simulink model "sedemo_async_clocks"  (Simulink 7.5)
settings: Solver=VariableStepDiscrete  StartTime=0.0  StopTime=10.0  MaxStep=inf  RelTol=1e-3
libraries: simulink x4, simeventstranslate1 x2, simeventsinfo x1, simeventssink1 x1
settings Model: Creator=The MathWorks Inc.  ExtModeAutoUpdateStatusClock=off
settings DataIOCC: SaveOutput=off  SaveTime=off
settings OptimizationCC: InitFltsAndDblsToZero=on
settings DebuggingCC: ReadBeforeWriteMsg=DisableAll  WriteAfterWriteMsg=DisableAll  WriteAfterReadMsg=DisableAll  AlgebraicLoopMsg=error  SolverPrmCheckMsg=none  StrictBusMsg=Warning
settings SimEventsCC: propDiagAttribOutput=1  propDiagFcnCallOutput=1  propDiagStatOutput=0

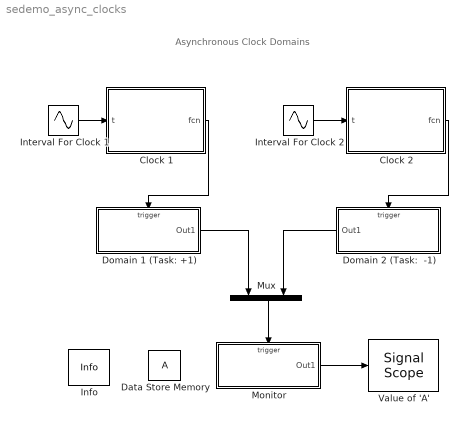
== system sedemo_async_clocks ==
  note: Asynchronous Clock Domains
  Clock 1 : Subsystem
  Clock 2 : Subsystem
  Data Store Memory : DataStoreMemory  DataStoreName=A  ReadBeforeWriteMsg=warning  WriteAfterWriteMsg=warning  WriteAfterReadMsg=warning  OutDataType=sfix(16)  OutScaling=2^0
  Domain 1 (Task: +1) : Subsystem  TreatAsAtomicUnit=on
  Domain 2 (Task:  -1) : Subsystem  TreatAsAtomicUnit=on
  Info : simeventsinfo/Info  SystemSampleTime=-1
  Interval For Clock 1 : Sin  Amplitude=-0.0001  Bias=.01  Frequency=1  Phase=pi/2  Samples=10  SampleTime=0  Offset=0
  Interval For Clock 2 : Sin  Amplitude=0.0001  Bias=.01  Frequency=1  Phase=pi/2  Samples=10  SampleTime=0  Offset=0
  Monitor : Subsystem  TreatAsAtomicUnit=on
      settings: PropExecContextOutsideSubsystem=on
  Mux : Mux  Inputs=2
  Value of 'A' : simeventssink1/Signal Scope  Priority=1  SystemSampleTime=-1  PlotType=Stair  InputType=Signal  NumInputs=1  AttributeNameY=Count  XInputOptionSignal=Event time  XInputOptionEntity=Event time  AttributeNameX=Count  EnableEntityOutport=on  XMin=-0.0999478213651573  XMax=10.0947299578809  XLimitExceededOption=Stretch axis limits  YLimitExceededOption=Stretch axis limits  AxisGrid=on  AxisLegend=off  LineDisables=""  LineColors=b  LineStyles=-  LineMarkers=.  OpenScopeAtSimStart=on  Title=Value of 'A': Clocks with Independent Drift  YLabel='A'  XLabel=Time  FigurePosition=[425 745 445 220]  AxisZoom=off  DataStoreOption=Limited  DataPointsLimit=10000  StatNumberArrived=Off  ShowCountPlotted=off  ShowToolbar=on
      settings: YMin=-2.05  YMax=3.05
  wires:
  Interval For Clock 1/1 -> Clock 1/1(t)
  Clock 1/1(fcn) -> Domain 1 (Task: +1)/Trigger
  Interval For Clock 2/1 -> Clock 2/1(t)
  Clock 2/1(fcn) -> Domain 2 (Task:  -1)/Trigger
  Domain 1 (Task: +1)/1(Out1) -> Mux/1
  Domain 2 (Task:  -1)/1(Out1) -> Mux/2
  Mux/1 -> Monitor/Trigger
  Monitor/1(Out1) -> Value of 'A'/1

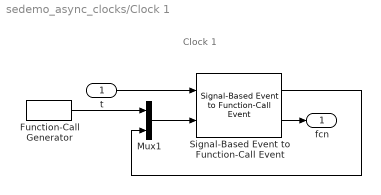
== system sedemo_async_clocks/Clock 1 ==
  note: Clock 1
  t : Inport
  Function-Call Generator : simulink/Ports & Subsystems/Function-Call Generator  sample_time=10000  numberOfIterations=1
  Mux1 : Mux  Inputs=2
  Signal-Based Event to Function-Call Event : simeventstranslate1/Signal-Based Event to Function-Call Event  Priority=1  SystemSampleTime=-1  GenerateFunctionCallUpon=Function call from port fcn  SignalEdgeOption=Rising  EnableE1Port=off  EnableF2Port=on  EnableE2Port=off  SpecifyEventPriority=on  PriorityFunctionCall=200  FunctionCallDelayFrom=Signal port t  DelayFunctionCall=0  StatNumberF1Calls=Off  StatNumberF2Calls=Off  MaskBlockType=none
  fcn : Outport
  wires:
  Mux1/1 -> Signal-Based Event to Function-Call Event/2
  Function-Call Generator/1 -> Mux1/1
  Signal-Based Event to Function-Call Event/1 -> Mux1/2
  t/1 -> Signal-Based Event to Function-Call Event/1
  Signal-Based Event to Function-Call Event/2 -> fcn/1

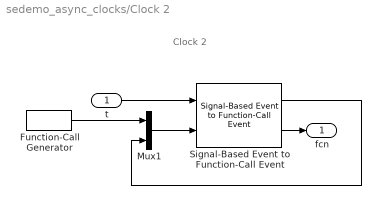
== system sedemo_async_clocks/Clock 2 ==
  note: Clock 2
  t : Inport
  Function-Call Generator : simulink/Ports & Subsystems/Function-Call Generator  sample_time=10000  numberOfIterations=1
  Mux1 : Mux  Inputs=2
  Signal-Based Event to Function-Call Event : simeventstranslate1/Signal-Based Event to Function-Call Event  Priority=1  SystemSampleTime=-1  GenerateFunctionCallUpon=Function call from port fcn  SignalEdgeOption=Rising  EnableE1Port=off  EnableF2Port=on  EnableE2Port=off  SpecifyEventPriority=on  PriorityFunctionCall=200  FunctionCallDelayFrom=Signal port t  DelayFunctionCall=0  StatNumberF1Calls=Off  StatNumberF2Calls=Off  MaskBlockType=none
  fcn : Outport
  wires:
  Mux1/1 -> Signal-Based Event to Function-Call Event/2
  Function-Call Generator/1 -> Mux1/1
  Signal-Based Event to Function-Call Event/1 -> Mux1/2
  t/1 -> Signal-Based Event to Function-Call Event/1
  Signal-Based Event to Function-Call Event/2 -> fcn/1

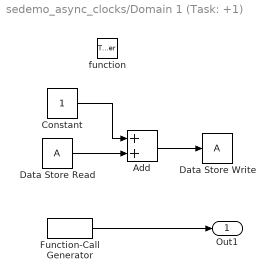
== system sedemo_async_clocks/Domain 1 (Task: +1) ==
  function : TriggerPort  TriggerType=function-call
  Add : Sum  OutDataType=sfix(16)  OutScaling=2^-10
  Constant : Constant  OutDataType=sfix(16)  OutScaling=2^0
  Data Store Read : DataStoreRead  DataStoreName=A  SampleTime=-1
  Data Store Write : DataStoreWrite  DataStoreName=A  SampleTime=-1
  Function-Call Generator : simulink/Ports & Subsystems/Function-Call Generator  sample_time=-1  numberOfIterations=1
  Out1 : Outport  OutDataType=sfix(16)  OutScaling=2^0
  wires:
  Add/1 -> Data Store Write/1
  Constant/1 -> Add/1
  Data Store Read/1 -> Add/2
  Function-Call Generator/1 -> Out1/1

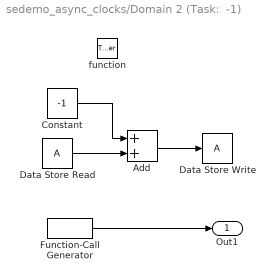
== system sedemo_async_clocks/Domain 2 (Task:  -1) ==
  function : TriggerPort  TriggerType=function-call
  Add : Sum  OutDataType=sfix(16)  OutScaling=2^-10
  Constant : Constant  Value=-1  OutDataType=sfix(16)  OutScaling=2^0
  Data Store Read : DataStoreRead  DataStoreName=A  SampleTime=-1
  Data Store Write : DataStoreWrite  DataStoreName=A  SampleTime=-1
  Function-Call Generator : simulink/Ports & Subsystems/Function-Call Generator  sample_time=-1  numberOfIterations=1
  Out1 : Outport  OutDataType=sfix(16)  OutScaling=2^0
  wires:
  Add/1 -> Data Store Write/1
  Constant/1 -> Add/1
  Data Store Read/1 -> Add/2
  Function-Call Generator/1 -> Out1/1

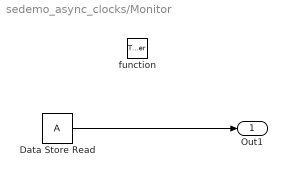
== system sedemo_async_clocks/Monitor ==
  function : TriggerPort  TriggerType=function-call
  Data Store Read : DataStoreRead  DataStoreName=A  SampleTime=-1
  Out1 : Outport  OutDataType=sfix(16)  OutScaling=2^0
  wires:
  Data Store Read/1 -> Out1/1
